simulink model "Engine_Control"  (R2016b)
settings: Solver=FixedStepDiscrete  StartTime=0  StopTime=inf  FixedStep=EngCtrl.tiSimnTiStep_C  RelTol=1e-3  EnableMultiTasking=on
settings Model: Creator=djuenema  LastModifiedBy=bunver
settings DataIOCC: SaveFormat=StructureWithTime  SaveOutput=off  DSMLogging=off  VisualizeSimOutput=off  SaveTime=off  SignalLoggingName=Results
settings OptimizationCC: BlockReduction=off  ConditionallyExecuteInputs=off  LifeSpan=inf
settings DebuggingCC: AllowSymbolicDim=off  SFUnexpectedBacktrackingDiag=warning  SFNoUnconditionalDefaultTransitionDiag=warning  SFExecutionAtInitializationDiag=none
settings ModelReferenceCC: ModelReferenceNumInstancesAllowed=Single  PropagateSignalLabelsOutOfModel=off
settings GRTTargetCC: TargetLangStandard=C89/C90 (ANSI)
settings ConfigComp: CovMetricSettings=dw  CovHtmlReporting=on  CovSaveCumulativeToWorkspaceVar=on  CovSaveSingleToWorkspaceVar=on  CovExternalEMLEnable=off

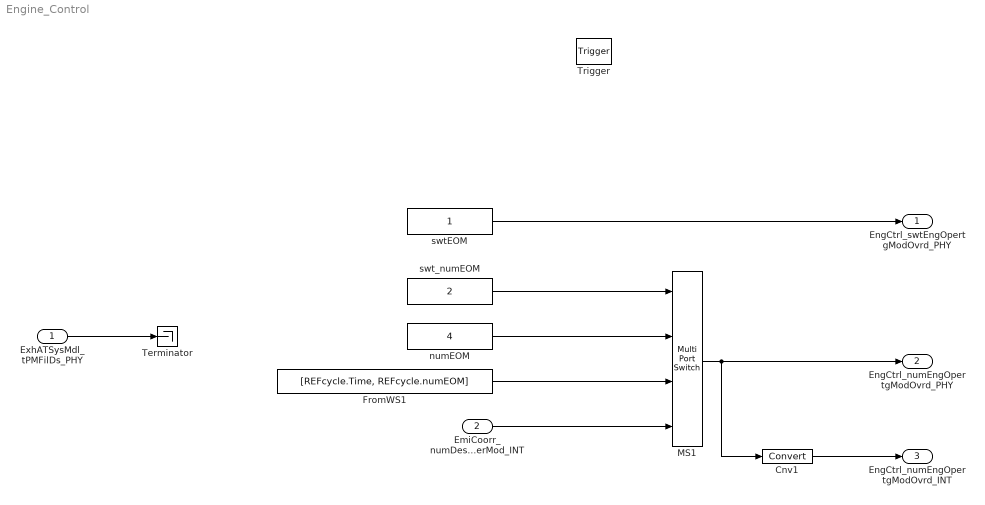
== system Engine_Control ==
  ExhATSysMdl_tPMFilDs_PHY : Inport
  EmiCoorr_numDesEngOperMod_INT : Inport  Port=2
  Trigger : TriggerPort  TriggerType=function-call  VariantControl=Variant  PortDimensions=1
  Cnv1 : DataTypeConversion
  FromWS1 : FromWorkspace  VariableName=[REFcycle.Time, REFcycle.numEOM]  Interpolate=off  OutputAfterFinalValue=Holding final value
  MS1 : MultiPortSwitch
  Terminator : Terminator
  numEOM : Constant  Value=4  SampleTime=-1
  swtEOM : Constant  SampleTime=-1
  swt_numEOM : Constant  Value=2  SampleTime=-1
  EngCtrl_swtEngOpertgModOvrd_PHY : Outport
  EngCtrl_numEngOpertgModOvrd_PHY : Outport  Port=2
  EngCtrl_numEngOpertgModOvrd_INT : Outport  Port=3
  wires:
  swtEOM/1 -> EngCtrl_swtEngOpertgModOvrd_PHY/1
  ExhATSysMdl_tPMFilDs_PHY/1 -> Terminator/1
  MS1/1 -> EngCtrl_numEngOpertgModOvrd_PHY/1, Cnv1/1
  numEOM/1 -> MS1/2
  swt_numEOM/1 -> MS1/1
  FromWS1/1 -> MS1/3
  EmiCoorr_numDesEngOperMod_INT/1 -> MS1/4
  Cnv1/1 -> EngCtrl_numEngOpertgModOvrd_INT/1
